simulink model "DSBsc_demodulation"  (R2019b)
settings: Solver=VariableStepAuto  StartTime=0.0  StopTime=0.008  RelTol=1e-3
libraries: dsparch4 x1
settings Model: Creator=Lenovo  LastModifiedBy=Lenovo

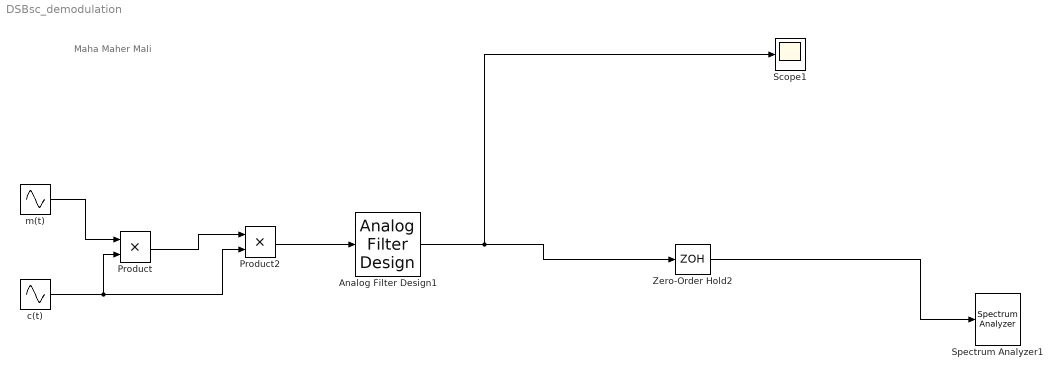
== system DSBsc_demodulation ==
  note: Maha Maher Mali
  Analog Filter Design1 : dsparch4/Analog Filter Design  method=Butterworth  filttype=Lowpass  N=8  Wlo=2*pi*1000*1.2  Whi=80  Rp=2  Rs=40
  Product : Product
  Product2 : Product
  Scope1 : Scope
  Spectrum Analyzer1 : SpectrumAnalyzer
  Zero-Order Hold2 : ZeroOrderHold  SampleTime=1/(10*1e3)
  c(t) : Sin  Frequency=2*pi*15000  SampleTime=0
  m(t) : Sin  Amplitude=0.85  Frequency=2*pi*1000  SampleTime=0
  wires:
  m(t)/1 -> Product/1
  Zero-Order Hold2/1 -> Spectrum Analyzer1/1
  Product/1 -> Product2/1
  c(t)/1 -> Product2/2, Product/2
  Product2/1 -> Analog Filter Design1/1
  Analog Filter Design1/1 -> Scope1/1, Zero-Order Hold2/1
